simulink model "DSR_delay_beta_test"  (R2021a)
settings: Solver=VariableStepAuto  StartTime=0.0  StopTime=10  RelTol=1e-3
values from neighbouring files (symbols this model uses):
  a = 0    [gainMaxDef.m]    (also in plot2.m = 2; simulink_test.m = 5)
  alpha = 1.195    [gainMaxDef.m]    (also in plot2.m = 1.9; simulink_test.m = 1.192)
  betac = 2    [plot2.m]    (also in simulink_test.m = 10)
  c1 = 1    [simulink_test.m]
  delay = 0.5    [plot2.m]    (also in simulink_test.m = 0.015)
  delay_a = 0.150    (= 0.15)    [plot2.m]    (also in simulink_test.m = 0.01)
  gnet = 40    [plot2.m]    (also in simulink_test.m = gnetset(k))
  omega = omegalist(l)    [gainMaxDef.m]    (also in plot2.m = 300; simulink_test.m = 0.8)
  omegader = 80    [simulink_test.m]
undefined symbols (not defined in the file or in its folder): betacd
libraries: cstblocks x37, simulink x4
(part 3 of 3)

== system DSR_delay_beta_test/DSR_Input2/(I-beta*K)V_dot_est/DerivativeEstimate ==
  pos : Inport
  pos1 : Inport  Port=2
  pos2 : Inport  Port=3
  pos3 : Inport  Port=4
  pos4 : Inport  Port=5
  pos5 : Inport  Port=6
  Derivative Estimator : Subsystem
  Derivative Estimator1 : Subsystem
  Derivative Estimator2 : Subsystem
  Derivative Estimator3 : Subsystem
  Derivative Estimator4 : Subsystem
  Derivative Estimator5 : Subsystem
  est : Outport
  est1 : Outport  Port=2
  est2 : Outport  Port=3
  est3 : Outport  Port=4
  est4 : Outport  Port=5
  est5 : Outport  Port=6
  wires:
  pos3/1 -> Derivative Estimator3/1(pos)
  Derivative Estimator4/1(est) -> est4/1
  Derivative Estimator2/1(est) -> est2/1
  Derivative Estimator3/1(est) -> est3/1
  Derivative Estimator1/1(est) -> est1/1
  pos1/1 -> Derivative Estimator1/1(pos)
  Derivative Estimator5/1(est) -> est5/1
  Derivative Estimator/1(est) -> est/1
  pos/1 -> Derivative Estimator/1(pos)
  pos2/1 -> Derivative Estimator2/1(pos)
  pos5/1 -> Derivative Estimator5/1(pos)
  pos4/1 -> Derivative Estimator4/1(pos)

== system DSR_delay_beta_test/DSR_Input2/(I-beta*K)V_dot_est/DerivativeEstimate1 ==
  pos : Inport
  pos1 : Inport  Port=2
  pos2 : Inport  Port=3
  pos3 : Inport  Port=4
  pos4 : Inport  Port=5
  pos5 : Inport  Port=6
  Derivative Estimator : Subsystem
  Derivative Estimator1 : Subsystem
  Derivative Estimator2 : Subsystem
  Derivative Estimator3 : Subsystem
  Derivative Estimator4 : Subsystem
  Derivative Estimator5 : Subsystem
  est : Outport
  est1 : Outport  Port=2
  est2 : Outport  Port=3
  est3 : Outport  Port=4
  est4 : Outport  Port=5
  est5 : Outport  Port=6
  wires:
  pos3/1 -> Derivative Estimator3/1(pos)
  Derivative Estimator4/1(est) -> est4/1
  Derivative Estimator2/1(est) -> est2/1
  Derivative Estimator3/1(est) -> est3/1
  Derivative Estimator1/1(est) -> est1/1
  pos1/1 -> Derivative Estimator1/1(pos)
  Derivative Estimator5/1(est) -> est5/1
  Derivative Estimator/1(est) -> est/1
  pos/1 -> Derivative Estimator/1(pos)
  pos2/1 -> Derivative Estimator2/1(pos)
  pos5/1 -> Derivative Estimator5/1(pos)
  pos4/1 -> Derivative Estimator4/1(pos)

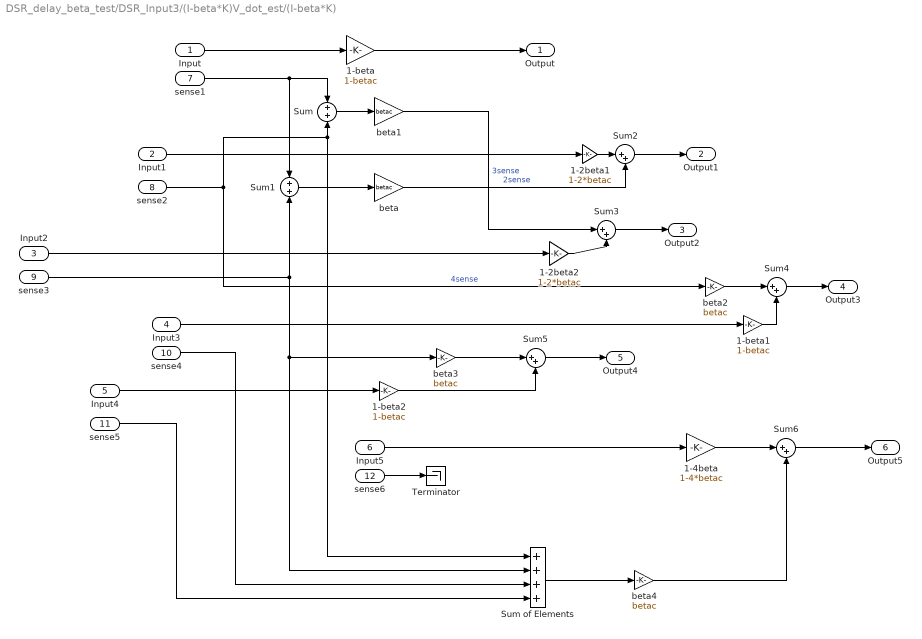
== system DSR_delay_beta_test/DSR_Input3/(I-beta*K)V_dot_est/(I-beta*K) ==
  Input : Inport
  Input1 : Inport  Port=2
  Input2 : Inport  Port=3
  Input3 : Inport  Port=4
  Input4 : Inport  Port=5
  Input5 : Inport  Port=6
  sense1 : Inport  Port=7
  sense2 : Inport  Port=8
  sense3 : Inport  Port=9
  sense4 : Inport  Port=10
  sense5 : Inport  Port=11
  sense6 : Inport  Port=12
  1-2beta1 : Gain  Gain=1-2*betac
  1-2beta2 : Gain  Gain=1-2*betac
  1-4beta : Gain  Gain=1-4*betac
  1-beta : Gain  Gain=1-betac
  1-beta1 : Gain  Gain=1-betac
  1-beta2 : Gain  Gain=1-betac
  Sum : Sum  Inputs=+|+
  Sum of Elements : Sum  Inputs=++++
  Sum1 : Sum  Inputs=+|+
  Sum{2..6} (5 alike) : Sum  Inputs=|++
  Terminator : Terminator
  beta{,1..4} (5 alike) : Gain  Gain=betac
  Output : Outport
  Output1 : Outport  Port=2
  Output2 : Outport  Port=3
  Output3 : Outport  Port=4
  Output4 : Outport  Port=5
  Output5 : Outport  Port=6
  wires:
  Input/1 -> 1-beta/1
  1-2beta2/1 -> Sum3/2
  1-beta2/1 -> Sum5/2
  Sum4/1 -> Output3/1
  1-beta/1 -> Output/1
  beta/1 -> Sum2/2  "2sense"
  Sum6/1 -> Output5/1
  1-beta1/1 -> Sum4/2
  Input2/1 -> 1-2beta2/1
  1-2beta1/1 -> Sum2/1
  Input1/1 -> 1-2beta1/1
  beta4/1 -> Sum6/2
  Sum/1 -> beta1/1
  Input3/1 -> 1-beta1/1
  beta3/1 -> Sum5/1
  beta1/1 -> Sum3/1  "3sense"
  beta2/1 -> Sum4/1
  Sum5/1 -> Output4/1
  Input4/1 -> 1-beta2/1
  Sum1/1 -> beta/1
  1-4beta/1 -> Sum6/1
  Sum2/1 -> Output1/1
  Sum3/1 -> Output2/1
  Input5/1 -> 1-4beta/1
  Sum of Elements/1 -> beta4/1
  sense1/1 -> Sum1/1, Sum/1
  sense2/1 -> beta2/1, Sum of Elements/1, Sum/2  "4sense"
  sense3/1 -> beta3/1, Sum of Elements/2, Sum1/2
  sense5/1 -> Sum of Elements/4
  sense4/1 -> Sum of Elements/3
  sense6/1 -> Terminator/1

== system DSR_delay_beta_test/DSR_Input3/(I-beta*K)V_dot_est/DerivativeEstimate ==
  pos : Inport
  pos1 : Inport  Port=2
  pos2 : Inport  Port=3
  pos3 : Inport  Port=4
  pos4 : Inport  Port=5
  pos5 : Inport  Port=6
  DSRdelayV1 : Subsystem
  DSRdelayV2 : Subsystem
  DSRdelayV3 : Subsystem
  DSRdelayV4 : Subsystem
  DSRdelayV5 : Subsystem
  DSRdelayV6 : Subsystem
  est : Outport
  est1 : Outport  Port=2
  est2 : Outport  Port=3
  est3 : Outport  Port=4
  est4 : Outport  Port=5
  est5 : Outport  Port=6
  wires:
  pos1/1 -> DSRdelayV1/1(Input)
  pos/1 -> DSRdelayV2/1(Input)
  DSRdelayV2/1(est) -> est/1
  pos2/1 -> DSRdelayV3/1(Input)
  pos3/1 -> DSRdelayV4/1(Input)
  pos4/1 -> DSRdelayV5/1(Input)
  pos5/1 -> DSRdelayV6/1(Input)
  DSRdelayV5/1(est) -> est4/1
  DSRdelayV6/1(est) -> est5/1
  DSRdelayV4/1(est) -> est3/1
  DSRdelayV3/1(est) -> est2/1
  DSRdelayV1/1(est) -> est1/1

== system DSR_delay_beta_test/DSR_Input3/(I-beta*K)V_dot_est/DerivativeEstimate1 ==
  pos : Inport
  pos1 : Inport  Port=2
  pos2 : Inport  Port=3
  pos3 : Inport  Port=4
  pos4 : Inport  Port=5
  pos5 : Inport  Port=6
  DSRdelayV1 : Subsystem
  DSRdelayV2 : Subsystem
  DSRdelayV3 : Subsystem
  DSRdelayV4 : Subsystem
  DSRdelayV5 : Subsystem
  DSRdelayV6 : Subsystem
  est : Outport
  est1 : Outport  Port=2
  est2 : Outport  Port=3
  est3 : Outport  Port=4
  est4 : Outport  Port=5
  est5 : Outport  Port=6
  wires:
  pos1/1 -> DSRdelayV1/1(Input)
  pos/1 -> DSRdelayV2/1(Input)
  DSRdelayV2/1(est) -> est/1
  pos2/1 -> DSRdelayV3/1(Input)
  pos3/1 -> DSRdelayV4/1(Input)
  pos4/1 -> DSRdelayV5/1(Input)
  pos5/1 -> DSRdelayV6/1(Input)
  DSRdelayV5/1(est) -> est4/1
  DSRdelayV6/1(est) -> est5/1
  DSRdelayV4/1(est) -> est3/1
  DSRdelayV3/1(est) -> est2/1
  DSRdelayV1/1(est) -> est1/1

== system DSR_delay_beta_test/DSR_Input1/(I-beta*K)V_dot_est/DerivativeEstimate/DSRdelayV1 ==
  Input : Inport
  Gain : Gain  Gain=1/delay
  Gain1 : Gain  Gain=1/delay
  Sum : Sum  Inputs=-+|
  Sum13 : Sum  Inputs=-+|
  Transfer Fcn : TransferFcn  Numerator=[omega]  Denominator=[1 omega]
  Transfer Fcn1 : TransferFcn  Numerator=[omega]  Denominator=[1 omega]
  Transport Delay : TransportDelay  DelayTime=delay
  Transport Delay13 : TransportDelay  DelayTime=delay
  est : Outport
  wires:
  Sum/1 -> Gain/1
  Gain/1 -> Transfer Fcn/1
  Transfer Fcn/1 -> Transport Delay13/1, Sum13/2
  Input/1 -> Transport Delay/1, Sum/2
  Transport Delay/1 -> Sum/1
  Transfer Fcn1/1 -> est/1
  Transport Delay13/1 -> Sum13/1
  Gain1/1 -> Transfer Fcn1/1
  Sum13/1 -> Gain1/1

== system DSR_delay_beta_test/DSR_Input1/(I-beta*K)V_dot_est/DerivativeEstimate/DSRdelayV2 ==
  Input : Inport
  Gain : Gain  Gain=1/delay
  Gain1 : Gain  Gain=1/delay
  Sum : Sum  Inputs=-+|
  Sum13 : Sum  Inputs=-+|
  Transfer Fcn : TransferFcn  Numerator=[omega]  Denominator=[1 omega]
  Transfer Fcn1 : TransferFcn  Numerator=[omega]  Denominator=[1 omega]
  Transport Delay : TransportDelay  DelayTime=delay
  Transport Delay13 : TransportDelay  DelayTime=delay
  est : Outport
  wires:
  Sum/1 -> Gain/1
  Gain/1 -> Transfer Fcn/1
  Transfer Fcn/1 -> Transport Delay13/1, Sum13/2
  Input/1 -> Transport Delay/1, Sum/2
  Transport Delay/1 -> Sum/1
  Transfer Fcn1/1 -> est/1
  Transport Delay13/1 -> Sum13/1
  Gain1/1 -> Transfer Fcn1/1
  Sum13/1 -> Gain1/1

== system DSR_delay_beta_test/DSR_Input1/(I-beta*K)V_dot_est/DerivativeEstimate/DSRdelayV3 ==
  Input : Inport
  Gain : Gain  Gain=1/delay
  Gain1 : Gain  Gain=1/delay
  Sum : Sum  Inputs=-+|
  Sum13 : Sum  Inputs=-+|
  Transfer Fcn : TransferFcn  Numerator=[omega]  Denominator=[1 omega]
  Transfer Fcn1 : TransferFcn  Numerator=[omega]  Denominator=[1 omega]
  Transport Delay : TransportDelay  DelayTime=delay
  Transport Delay13 : TransportDelay  DelayTime=delay
  est : Outport
  wires:
  Sum/1 -> Gain/1
  Gain/1 -> Transfer Fcn/1
  Transfer Fcn/1 -> Transport Delay13/1, Sum13/2
  Input/1 -> Transport Delay/1, Sum/2
  Transport Delay/1 -> Sum/1
  Transfer Fcn1/1 -> est/1
  Transport Delay13/1 -> Sum13/1
  Gain1/1 -> Transfer Fcn1/1
  Sum13/1 -> Gain1/1

== system DSR_delay_beta_test/DSR_Input1/(I-beta*K)V_dot_est/DerivativeEstimate/DSRdelayV4 ==
  Input : Inport
  Gain : Gain  Gain=1/delay
  Gain1 : Gain  Gain=1/delay
  Sum : Sum  Inputs=-+|
  Sum13 : Sum  Inputs=-+|
  Transfer Fcn : TransferFcn  Numerator=[omega]  Denominator=[1 omega]
  Transfer Fcn1 : TransferFcn  Numerator=[omega]  Denominator=[1 omega]
  Transport Delay : TransportDelay  DelayTime=delay
  Transport Delay13 : TransportDelay  DelayTime=delay
  est : Outport
  wires:
  Sum/1 -> Gain/1
  Gain/1 -> Transfer Fcn/1
  Transfer Fcn/1 -> Transport Delay13/1, Sum13/2
  Input/1 -> Transport Delay/1, Sum/2
  Transport Delay/1 -> Sum/1
  Transfer Fcn1/1 -> est/1
  Transport Delay13/1 -> Sum13/1
  Gain1/1 -> Transfer Fcn1/1
  Sum13/1 -> Gain1/1

== system DSR_delay_beta_test/DSR_Input1/(I-beta*K)V_dot_est/DerivativeEstimate/DSRdelayV5 ==
  Input : Inport
  Gain : Gain  Gain=1/delay
  Gain1 : Gain  Gain=1/delay
  Sum : Sum  Inputs=-+|
  Sum13 : Sum  Inputs=-+|
  Transfer Fcn : TransferFcn  Numerator=[omega]  Denominator=[1 omega]
  Transfer Fcn1 : TransferFcn  Numerator=[omega]  Denominator=[1 omega]
  Transport Delay : TransportDelay  DelayTime=delay
  Transport Delay13 : TransportDelay  DelayTime=delay
  est : Outport
  wires:
  Sum/1 -> Gain/1
  Gain/1 -> Transfer Fcn/1
  Transfer Fcn/1 -> Transport Delay13/1, Sum13/2
  Input/1 -> Transport Delay/1, Sum/2
  Transport Delay/1 -> Sum/1
  Transfer Fcn1/1 -> est/1
  Transport Delay13/1 -> Sum13/1
  Gain1/1 -> Transfer Fcn1/1
  Sum13/1 -> Gain1/1

== system DSR_delay_beta_test/DSR_Input1/(I-beta*K)V_dot_est/DerivativeEstimate/DSRdelayV6 ==
  Input : Inport
  Gain : Gain  Gain=1/delay
  Gain1 : Gain  Gain=1/delay
  Sum : Sum  Inputs=-+|
  Sum13 : Sum  Inputs=-+|
  Transfer Fcn : TransferFcn  Numerator=[omega]  Denominator=[1 omega]
  Transfer Fcn1 : TransferFcn  Numerator=[omega]  Denominator=[1 omega]
  Transport Delay : TransportDelay  DelayTime=delay
  Transport Delay13 : TransportDelay  DelayTime=delay
  est : Outport
  wires:
  Sum/1 -> Gain/1
  Gain/1 -> Transfer Fcn/1
  Transfer Fcn/1 -> Transport Delay13/1, Sum13/2
  Input/1 -> Transport Delay/1, Sum/2
  Transport Delay/1 -> Sum/1
  Transfer Fcn1/1 -> est/1
  Transport Delay13/1 -> Sum13/1
  Gain1/1 -> Transfer Fcn1/1
  Sum13/1 -> Gain1/1

== system DSR_delay_beta_test/DSR_Input1/(I-beta*K)V_dot_est/DerivativeEstimate1/DSRdelayV1 ==
  Input : Inport
  Gain : Gain  Gain=1/delay
  Gain1 : Gain  Gain=1/delay
  Sum : Sum  Inputs=-+|
  Sum13 : Sum  Inputs=-+|
  Transfer Fcn : TransferFcn  Numerator=[omega]  Denominator=[1 omega]
  Transfer Fcn1 : TransferFcn  Numerator=[omega]  Denominator=[1 omega]
  Transport Delay : TransportDelay  DelayTime=delay
  Transport Delay13 : TransportDelay  DelayTime=delay
  est : Outport
  wires:
  Sum/1 -> Gain/1
  Gain/1 -> Transfer Fcn/1
  Transfer Fcn/1 -> Transport Delay13/1, Sum13/2
  Input/1 -> Transport Delay/1, Sum/2
  Transport Delay/1 -> Sum/1
  Transfer Fcn1/1 -> est/1
  Transport Delay13/1 -> Sum13/1
  Gain1/1 -> Transfer Fcn1/1
  Sum13/1 -> Gain1/1

== system DSR_delay_beta_test/DSR_Input1/(I-beta*K)V_dot_est/DerivativeEstimate1/DSRdelayV2 ==
  Input : Inport
  Gain : Gain  Gain=1/delay
  Gain1 : Gain  Gain=1/delay
  Scope : Scope  NumInputPorts=5
  Sum : Sum  Inputs=-+|
  Sum13 : Sum  Inputs=-+|
  Transfer Fcn : TransferFcn  Numerator=[omega]  Denominator=[1 omega]
  Transfer Fcn1 : TransferFcn  Numerator=[omega]  Denominator=[1 omega]
  Transport Delay : TransportDelay  DelayTime=delay
  Transport Delay13 : TransportDelay  DelayTime=delay
  est : Outport
  wires:
  Sum/1 -> Gain/1
  Gain/1 -> Scope/2, Transfer Fcn/1
  Transfer Fcn/1 -> Transport Delay13/1, Sum13/2, Scope/3
  Input/1 -> Transport Delay/1, Scope/1, Sum/2
  Transport Delay/1 -> Sum/1
  Transfer Fcn1/1 -> Scope/5, est/1
  Transport Delay13/1 -> Sum13/1
  Gain1/1 -> Scope/4, Transfer Fcn1/1
  Sum13/1 -> Gain1/1

== system DSR_delay_beta_test/DSR_Input1/(I-beta*K)V_dot_est/DerivativeEstimate1/DSRdelayV3 ==
  Input : Inport
  Gain : Gain  Gain=1/delay
  Gain1 : Gain  Gain=1/delay
  Sum : Sum  Inputs=-+|
  Sum13 : Sum  Inputs=-+|
  Transfer Fcn : TransferFcn  Numerator=[omega]  Denominator=[1 omega]
  Transfer Fcn1 : TransferFcn  Numerator=[omega]  Denominator=[1 omega]
  Transport Delay : TransportDelay  DelayTime=delay
  Transport Delay13 : TransportDelay  DelayTime=delay
  est : Outport
  wires:
  Sum/1 -> Gain/1
  Gain/1 -> Transfer Fcn/1
  Transfer Fcn/1 -> Transport Delay13/1, Sum13/2
  Input/1 -> Transport Delay/1, Sum/2
  Transport Delay/1 -> Sum/1
  Transfer Fcn1/1 -> est/1
  Transport Delay13/1 -> Sum13/1
  Gain1/1 -> Transfer Fcn1/1
  Sum13/1 -> Gain1/1

== system DSR_delay_beta_test/DSR_Input1/(I-beta*K)V_dot_est/DerivativeEstimate1/DSRdelayV4 ==
  Input : Inport
  Gain : Gain  Gain=1/delay
  Gain1 : Gain  Gain=1/delay
  Sum : Sum  Inputs=-+|
  Sum13 : Sum  Inputs=-+|
  Transfer Fcn : TransferFcn  Numerator=[omega]  Denominator=[1 omega]
  Transfer Fcn1 : TransferFcn  Numerator=[omega]  Denominator=[1 omega]
  Transport Delay : TransportDelay  DelayTime=delay
  Transport Delay13 : TransportDelay  DelayTime=delay
  est : Outport
  wires:
  Sum/1 -> Gain/1
  Gain/1 -> Transfer Fcn/1
  Transfer Fcn/1 -> Transport Delay13/1, Sum13/2
  Input/1 -> Transport Delay/1, Sum/2
  Transport Delay/1 -> Sum/1
  Transfer Fcn1/1 -> est/1
  Transport Delay13/1 -> Sum13/1
  Gain1/1 -> Transfer Fcn1/1
  Sum13/1 -> Gain1/1

== system DSR_delay_beta_test/DSR_Input1/(I-beta*K)V_dot_est/DerivativeEstimate1/DSRdelayV5 ==
  Input : Inport
  Gain : Gain  Gain=1/delay
  Gain1 : Gain  Gain=1/delay
  Sum : Sum  Inputs=-+|
  Sum13 : Sum  Inputs=-+|
  Transfer Fcn : TransferFcn  Numerator=[omega]  Denominator=[1 omega]
  Transfer Fcn1 : TransferFcn  Numerator=[omega]  Denominator=[1 omega]
  Transport Delay : TransportDelay  DelayTime=delay
  Transport Delay13 : TransportDelay  DelayTime=delay
  est : Outport
  wires:
  Sum/1 -> Gain/1
  Gain/1 -> Transfer Fcn/1
  Transfer Fcn/1 -> Transport Delay13/1, Sum13/2
  Input/1 -> Transport Delay/1, Sum/2
  Transport Delay/1 -> Sum/1
  Transfer Fcn1/1 -> est/1
  Transport Delay13/1 -> Sum13/1
  Gain1/1 -> Transfer Fcn1/1
  Sum13/1 -> Gain1/1

== system DSR_delay_beta_test/DSR_Input1/(I-beta*K)V_dot_est/DerivativeEstimate1/DSRdelayV6 ==
  Input : Inport
  Gain : Gain  Gain=1/delay
  Gain1 : Gain  Gain=1/delay
  Sum : Sum  Inputs=-+|
  Sum13 : Sum  Inputs=-+|
  Transfer Fcn : TransferFcn  Numerator=[omega]  Denominator=[1 omega]
  Transfer Fcn1 : TransferFcn  Numerator=[omega]  Denominator=[1 omega]
  Transport Delay : TransportDelay  DelayTime=delay
  Transport Delay13 : TransportDelay  DelayTime=delay
  est : Outport
  wires:
  Sum/1 -> Gain/1
  Gain/1 -> Transfer Fcn/1
  Transfer Fcn/1 -> Transport Delay13/1, Sum13/2
  Input/1 -> Transport Delay/1, Sum/2
  Transport Delay/1 -> Sum/1
  Transfer Fcn1/1 -> est/1
  Transport Delay13/1 -> Sum13/1
  Gain1/1 -> Transfer Fcn1/1
  Sum13/1 -> Gain1/1

== system DSR_delay_beta_test/DSR_Input2/(I-beta*K)V_dot_est/DerivativeEstimate/Derivative Estimator ==
  pos : Inport
  DSRdelay : Subsystem
  LPF : TransferFcn  Numerator=[omega^2]  Denominator=[delay^2 2*omega*delay^2 omega^2*delay^2]
  est : Outport
  wires:
  LPF/1 -> DSRdelay/1(Input)
  DSRdelay/1(Out1) -> est/1
  pos/1 -> LPF/1

== system DSR_delay_beta_test/DSR_Input2/(I-beta*K)V_dot_est/DerivativeEstimate/Derivative Estimator1 ==
  pos : Inport
  DSRdelay : Subsystem
  LPF : TransferFcn  Numerator=[omega^2]  Denominator=[delay^2 2*omega*delay^2 omega^2*delay^2]
  est : Outport
  wires:
  LPF/1 -> DSRdelay/1(Input)
  DSRdelay/1(Out1) -> est/1
  pos/1 -> LPF/1

== system DSR_delay_beta_test/DSR_Input2/(I-beta*K)V_dot_est/DerivativeEstimate/Derivative Estimator2 ==
  pos : Inport
  DSRdelay : Subsystem
  LPF : TransferFcn  Numerator=[omega^2]  Denominator=[delay^2 2*omega*delay^2 omega^2*delay^2]
  est : Outport
  wires:
  LPF/1 -> DSRdelay/1(Input)
  DSRdelay/1(Out1) -> est/1
  pos/1 -> LPF/1

== system DSR_delay_beta_test/DSR_Input2/(I-beta*K)V_dot_est/DerivativeEstimate/Derivative Estimator3 ==
  pos : Inport
  DSRdelay : Subsystem
  LPF : TransferFcn  Numerator=[omega^2]  Denominator=[delay^2 2*omega*delay^2 omega^2*delay^2]
  est : Outport
  wires:
  LPF/1 -> DSRdelay/1(Input)
  DSRdelay/1(Out1) -> est/1
  pos/1 -> LPF/1

== system DSR_delay_beta_test/DSR_Input2/(I-beta*K)V_dot_est/DerivativeEstimate/Derivative Estimator4 ==
  pos : Inport
  DSRdelay : Subsystem
  LPF : TransferFcn  Numerator=[omega^2]  Denominator=[delay^2 2*omega*delay^2 omega^2*delay^2]
  est : Outport
  wires:
  LPF/1 -> DSRdelay/1(Input)
  DSRdelay/1(Out1) -> est/1
  pos/1 -> LPF/1

== system DSR_delay_beta_test/DSR_Input2/(I-beta*K)V_dot_est/DerivativeEstimate/Derivative Estimator5 ==
  pos : Inport
  DSRdelay : Subsystem
  LPF : TransferFcn  Numerator=[omega^2]  Denominator=[delay^2 2*omega*delay^2 omega^2*delay^2]
  est : Outport
  wires:
  LPF/1 -> DSRdelay/1(Input)
  DSRdelay/1(Out1) -> est/1
  pos/1 -> LPF/1

== system DSR_delay_beta_test/DSR_Input2/(I-beta*K)V_dot_est/DerivativeEstimate1/Derivative Estimator ==
  pos : Inport
  DSRdelay : Subsystem
  LPF : TransferFcn  Numerator=[omega^2]  Denominator=[delay^2 2*omega*delay^2 omega^2*delay^2]
  est : Outport
  wires:
  LPF/1 -> DSRdelay/1(Input)
  DSRdelay/1(Out1) -> est/1
  pos/1 -> LPF/1

== system DSR_delay_beta_test/DSR_Input2/(I-beta*K)V_dot_est/DerivativeEstimate1/Derivative Estimator1 ==
  pos : Inport
  DSRdelay : Subsystem
  LPF : TransferFcn  Numerator=[omega^2]  Denominator=[delay^2 2*omega*delay^2 omega^2*delay^2]
  est : Outport
  wires:
  LPF/1 -> DSRdelay/1(Input)
  DSRdelay/1(Out1) -> est/1
  pos/1 -> LPF/1

== system DSR_delay_beta_test/DSR_Input2/(I-beta*K)V_dot_est/DerivativeEstimate1/Derivative Estimator2 ==
  pos : Inport
  DSRdelay : Subsystem
  LPF : TransferFcn  Numerator=[omega^2]  Denominator=[delay^2 2*omega*delay^2 omega^2*delay^2]
  est : Outport
  wires:
  LPF/1 -> DSRdelay/1(Input)
  DSRdelay/1(Out1) -> est/1
  pos/1 -> LPF/1

== system DSR_delay_beta_test/DSR_Input2/(I-beta*K)V_dot_est/DerivativeEstimate1/Derivative Estimator3 ==
  pos : Inport
  DSRdelay : Subsystem
  LPF : TransferFcn  Numerator=[omega^2]  Denominator=[delay^2 2*omega*delay^2 omega^2*delay^2]
  est : Outport
  wires:
  LPF/1 -> DSRdelay/1(Input)
  DSRdelay/1(Out1) -> est/1
  pos/1 -> LPF/1

== system DSR_delay_beta_test/DSR_Input2/(I-beta*K)V_dot_est/DerivativeEstimate1/Derivative Estimator4 ==
  pos : Inport
  DSRdelay : Subsystem
  LPF : TransferFcn  Numerator=[omega^2]  Denominator=[delay^2 2*omega*delay^2 omega^2*delay^2]
  est : Outport
  wires:
  LPF/1 -> DSRdelay/1(Input)
  DSRdelay/1(Out1) -> est/1
  pos/1 -> LPF/1

== system DSR_delay_beta_test/DSR_Input2/(I-beta*K)V_dot_est/DerivativeEstimate1/Derivative Estimator5 ==
  pos : Inport
  DSRdelay : Subsystem
  LPF : TransferFcn  Numerator=[omega^2]  Denominator=[delay^2 2*omega*delay^2 omega^2*delay^2]
  est : Outport
  wires:
  LPF/1 -> DSRdelay/1(Input)
  DSRdelay/1(Out1) -> est/1
  pos/1 -> LPF/1

== system DSR_delay_beta_test/DSR_Input3/(I-beta*K)V_dot_est/DerivativeEstimate/DSRdelayV1 ==
  Input : Inport
  Gain : Gain  Gain=1/delay
  Gain1 : Gain  Gain=1/delay
  Sum : Sum  Inputs=-+|
  Sum13 : Sum  Inputs=-+|
  Transfer Fcn : TransferFcn  Numerator=[omega]  Denominator=[1 omega]
  Transfer Fcn1 : TransferFcn  Numerator=[omega]  Denominator=[1 omega]
  Transport Delay : TransportDelay  DelayTime=delay
  Transport Delay13 : TransportDelay  DelayTime=delay
  est : Outport
  wires:
  Sum/1 -> Gain/1
  Gain/1 -> Transfer Fcn/1
  Transfer Fcn/1 -> Transport Delay13/1, Sum13/2
  Input/1 -> Transport Delay/1, Sum/2
  Transport Delay/1 -> Sum/1
  Transfer Fcn1/1 -> est/1
  Transport Delay13/1 -> Sum13/1
  Gain1/1 -> Transfer Fcn1/1
  Sum13/1 -> Gain1/1

== system DSR_delay_beta_test/DSR_Input3/(I-beta*K)V_dot_est/DerivativeEstimate/DSRdelayV2 ==
  Input : Inport
  Gain : Gain  Gain=1/delay
  Gain1 : Gain  Gain=1/delay
  Sum : Sum  Inputs=-+|
  Sum13 : Sum  Inputs=-+|
  Transfer Fcn : TransferFcn  Numerator=[omega]  Denominator=[1 omega]
  Transfer Fcn1 : TransferFcn  Numerator=[omega]  Denominator=[1 omega]
  Transport Delay : TransportDelay  DelayTime=delay
  Transport Delay13 : TransportDelay  DelayTime=delay
  est : Outport
  wires:
  Sum/1 -> Gain/1
  Gain/1 -> Transfer Fcn/1
  Transfer Fcn/1 -> Transport Delay13/1, Sum13/2
  Input/1 -> Transport Delay/1, Sum/2
  Transport Delay/1 -> Sum/1
  Transfer Fcn1/1 -> est/1
  Transport Delay13/1 -> Sum13/1
  Gain1/1 -> Transfer Fcn1/1
  Sum13/1 -> Gain1/1

== system DSR_delay_beta_test/DSR_Input3/(I-beta*K)V_dot_est/DerivativeEstimate/DSRdelayV3 ==
  Input : Inport
  Gain : Gain  Gain=1/delay
  Gain1 : Gain  Gain=1/delay
  Sum : Sum  Inputs=-+|
  Sum13 : Sum  Inputs=-+|
  Transfer Fcn : TransferFcn  Numerator=[omega]  Denominator=[1 omega]
  Transfer Fcn1 : TransferFcn  Numerator=[omega]  Denominator=[1 omega]
  Transport Delay : TransportDelay  DelayTime=delay
  Transport Delay13 : TransportDelay  DelayTime=delay
  est : Outport
  wires:
  Sum/1 -> Gain/1
  Gain/1 -> Transfer Fcn/1
  Transfer Fcn/1 -> Transport Delay13/1, Sum13/2
  Input/1 -> Transport Delay/1, Sum/2
  Transport Delay/1 -> Sum/1
  Transfer Fcn1/1 -> est/1
  Transport Delay13/1 -> Sum13/1
  Gain1/1 -> Transfer Fcn1/1
  Sum13/1 -> Gain1/1

== system DSR_delay_beta_test/DSR_Input3/(I-beta*K)V_dot_est/DerivativeEstimate/DSRdelayV4 ==
  Input : Inport
  Gain : Gain  Gain=1/delay
  Gain1 : Gain  Gain=1/delay
  Sum : Sum  Inputs=-+|
  Sum13 : Sum  Inputs=-+|
  Transfer Fcn : TransferFcn  Numerator=[omega]  Denominator=[1 omega]
  Transfer Fcn1 : TransferFcn  Numerator=[omega]  Denominator=[1 omega]
  Transport Delay : TransportDelay  DelayTime=delay
  Transport Delay13 : TransportDelay  DelayTime=delay
  est : Outport
  wires:
  Sum/1 -> Gain/1
  Gain/1 -> Transfer Fcn/1
  Transfer Fcn/1 -> Transport Delay13/1, Sum13/2
  Input/1 -> Transport Delay/1, Sum/2
  Transport Delay/1 -> Sum/1
  Transfer Fcn1/1 -> est/1
  Transport Delay13/1 -> Sum13/1
  Gain1/1 -> Transfer Fcn1/1
  Sum13/1 -> Gain1/1

== system DSR_delay_beta_test/DSR_Input3/(I-beta*K)V_dot_est/DerivativeEstimate/DSRdelayV5 ==
  Input : Inport
  Gain : Gain  Gain=1/delay
  Gain1 : Gain  Gain=1/delay
  Sum : Sum  Inputs=-+|
  Sum13 : Sum  Inputs=-+|
  Transfer Fcn : TransferFcn  Numerator=[omega]  Denominator=[1 omega]
  Transfer Fcn1 : TransferFcn  Numerator=[omega]  Denominator=[1 omega]
  Transport Delay : TransportDelay  DelayTime=delay
  Transport Delay13 : TransportDelay  DelayTime=delay
  est : Outport
  wires:
  Sum/1 -> Gain/1
  Gain/1 -> Transfer Fcn/1
  Transfer Fcn/1 -> Transport Delay13/1, Sum13/2
  Input/1 -> Transport Delay/1, Sum/2
  Transport Delay/1 -> Sum/1
  Transfer Fcn1/1 -> est/1
  Transport Delay13/1 -> Sum13/1
  Gain1/1 -> Transfer Fcn1/1
  Sum13/1 -> Gain1/1

== system DSR_delay_beta_test/DSR_Input3/(I-beta*K)V_dot_est/DerivativeEstimate/DSRdelayV6 ==
  Input : Inport
  Gain : Gain  Gain=1/delay
  Gain1 : Gain  Gain=1/delay
  Sum : Sum  Inputs=-+|
  Sum13 : Sum  Inputs=-+|
  Transfer Fcn : TransferFcn  Numerator=[omega]  Denominator=[1 omega]
  Transfer Fcn1 : TransferFcn  Numerator=[omega]  Denominator=[1 omega]
  Transport Delay : TransportDelay  DelayTime=delay
  Transport Delay13 : TransportDelay  DelayTime=delay
  est : Outport
  wires:
  Sum/1 -> Gain/1
  Gain/1 -> Transfer Fcn/1
  Transfer Fcn/1 -> Transport Delay13/1, Sum13/2
  Input/1 -> Transport Delay/1, Sum/2
  Transport Delay/1 -> Sum/1
  Transfer Fcn1/1 -> est/1
  Transport Delay13/1 -> Sum13/1
  Gain1/1 -> Transfer Fcn1/1
  Sum13/1 -> Gain1/1

== system DSR_delay_beta_test/DSR_Input3/(I-beta*K)V_dot_est/DerivativeEstimate1/DSRdelayV1 ==
  Input : Inport
  Gain : Gain  Gain=1/delay
  Gain1 : Gain  Gain=1/delay
  Sum : Sum  Inputs=-+|
  Sum13 : Sum  Inputs=-+|
  Transfer Fcn : TransferFcn  Numerator=[omega]  Denominator=[1 omega]
  Transfer Fcn1 : TransferFcn  Numerator=[omega]  Denominator=[1 omega]
  Transport Delay : TransportDelay  DelayTime=delay
  Transport Delay13 : TransportDelay  DelayTime=delay
  est : Outport
  wires:
  Sum/1 -> Gain/1
  Gain/1 -> Transfer Fcn/1
  Transfer Fcn/1 -> Transport Delay13/1, Sum13/2
  Input/1 -> Transport Delay/1, Sum/2
  Transport Delay/1 -> Sum/1
  Transfer Fcn1/1 -> est/1
  Transport Delay13/1 -> Sum13/1
  Gain1/1 -> Transfer Fcn1/1
  Sum13/1 -> Gain1/1

== system DSR_delay_beta_test/DSR_Input3/(I-beta*K)V_dot_est/DerivativeEstimate1/DSRdelayV2 ==
  Input : Inport
  Gain : Gain  Gain=1/delay
  Gain1 : Gain  Gain=1/delay
  Scope : Scope  NumInputPorts=5
  Sum : Sum  Inputs=-+|
  Sum13 : Sum  Inputs=-+|
  Transfer Fcn : TransferFcn  Numerator=[omega]  Denominator=[1 omega]
  Transfer Fcn1 : TransferFcn  Numerator=[omega]  Denominator=[1 omega]
  Transport Delay : TransportDelay  DelayTime=delay
  Transport Delay13 : TransportDelay  DelayTime=delay
  est : Outport
  wires:
  Sum/1 -> Gain/1
  Gain/1 -> Scope/2, Transfer Fcn/1
  Transfer Fcn/1 -> Transport Delay13/1, Sum13/2, Scope/3
  Input/1 -> Transport Delay/1, Scope/1, Sum/2
  Transport Delay/1 -> Sum/1
  Transfer Fcn1/1 -> Scope/5, est/1
  Transport Delay13/1 -> Sum13/1
  Gain1/1 -> Scope/4, Transfer Fcn1/1
  Sum13/1 -> Gain1/1

== system DSR_delay_beta_test/DSR_Input3/(I-beta*K)V_dot_est/DerivativeEstimate1/DSRdelayV3 ==
  Input : Inport
  Gain : Gain  Gain=1/delay
  Gain1 : Gain  Gain=1/delay
  Sum : Sum  Inputs=-+|
  Sum13 : Sum  Inputs=-+|
  Transfer Fcn : TransferFcn  Numerator=[omega]  Denominator=[1 omega]
  Transfer Fcn1 : TransferFcn  Numerator=[omega]  Denominator=[1 omega]
  Transport Delay : TransportDelay  DelayTime=delay
  Transport Delay13 : TransportDelay  DelayTime=delay
  est : Outport
  wires:
  Sum/1 -> Gain/1
  Gain/1 -> Transfer Fcn/1
  Transfer Fcn/1 -> Transport Delay13/1, Sum13/2
  Input/1 -> Transport Delay/1, Sum/2
  Transport Delay/1 -> Sum/1
  Transfer Fcn1/1 -> est/1
  Transport Delay13/1 -> Sum13/1
  Gain1/1 -> Transfer Fcn1/1
  Sum13/1 -> Gain1/1

== system DSR_delay_beta_test/DSR_Input3/(I-beta*K)V_dot_est/DerivativeEstimate1/DSRdelayV4 ==
  Input : Inport
  Gain : Gain  Gain=1/delay
  Gain1 : Gain  Gain=1/delay
  Sum : Sum  Inputs=-+|
  Sum13 : Sum  Inputs=-+|
  Transfer Fcn : TransferFcn  Numerator=[omega]  Denominator=[1 omega]
  Transfer Fcn1 : TransferFcn  Numerator=[omega]  Denominator=[1 omega]
  Transport Delay : TransportDelay  DelayTime=delay
  Transport Delay13 : TransportDelay  DelayTime=delay
  est : Outport
  wires:
  Sum/1 -> Gain/1
  Gain/1 -> Transfer Fcn/1
  Transfer Fcn/1 -> Transport Delay13/1, Sum13/2
  Input/1 -> Transport Delay/1, Sum/2
  Transport Delay/1 -> Sum/1
  Transfer Fcn1/1 -> est/1
  Transport Delay13/1 -> Sum13/1
  Gain1/1 -> Transfer Fcn1/1
  Sum13/1 -> Gain1/1

== system DSR_delay_beta_test/DSR_Input3/(I-beta*K)V_dot_est/DerivativeEstimate1/DSRdelayV5 ==
  Input : Inport
  Gain : Gain  Gain=1/delay
  Gain1 : Gain  Gain=1/delay
  Sum : Sum  Inputs=-+|
  Sum13 : Sum  Inputs=-+|
  Transfer Fcn : TransferFcn  Numerator=[omega]  Denominator=[1 omega]
  Transfer Fcn1 : TransferFcn  Numerator=[omega]  Denominator=[1 omega]
  Transport Delay : TransportDelay  DelayTime=delay
  Transport Delay13 : TransportDelay  DelayTime=delay
  est : Outport
  wires:
  Sum/1 -> Gain/1
  Gain/1 -> Transfer Fcn/1
  Transfer Fcn/1 -> Transport Delay13/1, Sum13/2
  Input/1 -> Transport Delay/1, Sum/2
  Transport Delay/1 -> Sum/1
  Transfer Fcn1/1 -> est/1
  Transport Delay13/1 -> Sum13/1
  Gain1/1 -> Transfer Fcn1/1
  Sum13/1 -> Gain1/1

== system DSR_delay_beta_test/DSR_Input3/(I-beta*K)V_dot_est/DerivativeEstimate1/DSRdelayV6 ==
  Input : Inport
  Gain : Gain  Gain=1/delay
  Gain1 : Gain  Gain=1/delay
  Sum : Sum  Inputs=-+|
  Sum13 : Sum  Inputs=-+|
  Transfer Fcn : TransferFcn  Numerator=[omega]  Denominator=[1 omega]
  Transfer Fcn1 : TransferFcn  Numerator=[omega]  Denominator=[1 omega]
  Transport Delay : TransportDelay  DelayTime=delay
  Transport Delay13 : TransportDelay  DelayTime=delay
  est : Outport
  wires:
  Sum/1 -> Gain/1
  Gain/1 -> Transfer Fcn/1
  Transfer Fcn/1 -> Transport Delay13/1, Sum13/2
  Input/1 -> Transport Delay/1, Sum/2
  Transport Delay/1 -> Sum/1
  Transfer Fcn1/1 -> est/1
  Transport Delay13/1 -> Sum13/1
  Gain1/1 -> Transfer Fcn1/1
  Sum13/1 -> Gain1/1

== system DSR_delay_beta_test/DSR_Input2/(I-beta*K)V_dot_est/DerivativeEstimate/Derivative Estimator/DSRdelay ==
  Input : Inport
  Gain : Gain  Gain=2
  Sum : Sum  Inputs=-++
  Transport Delay1 : TransportDelay  DelayTime=2*delay
  Transport Delay2 : TransportDelay  DelayTime=delay
  Out1 : Outport
  wires:
  Input/1 -> Transport Delay2/1, Transport Delay1/1, Sum/2
  Transport Delay2/1 -> Gain/1
  Transport Delay1/1 -> Sum/3
  Gain/1 -> Sum/1
  Sum/1 -> Out1/1

== system DSR_delay_beta_test/DSR_Input2/(I-beta*K)V_dot_est/DerivativeEstimate/Derivative Estimator1/DSRdelay ==
  Input : Inport
  Gain : Gain  Gain=2
  Sum : Sum  Inputs=-++
  Transport Delay1 : TransportDelay  DelayTime=2*delay
  Transport Delay2 : TransportDelay  DelayTime=delay
  Out1 : Outport
  wires:
  Input/1 -> Transport Delay2/1, Transport Delay1/1, Sum/2
  Transport Delay2/1 -> Gain/1
  Transport Delay1/1 -> Sum/3
  Gain/1 -> Sum/1
  Sum/1 -> Out1/1

== system DSR_delay_beta_test/DSR_Input2/(I-beta*K)V_dot_est/DerivativeEstimate/Derivative Estimator2/DSRdelay ==
  Input : Inport
  Gain : Gain  Gain=2
  Sum : Sum  Inputs=-++
  Transport Delay1 : TransportDelay  DelayTime=2*delay
  Transport Delay2 : TransportDelay  DelayTime=delay
  Out1 : Outport
  wires:
  Input/1 -> Transport Delay2/1, Transport Delay1/1, Sum/2
  Transport Delay2/1 -> Gain/1
  Transport Delay1/1 -> Sum/3
  Gain/1 -> Sum/1
  Sum/1 -> Out1/1

== system DSR_delay_beta_test/DSR_Input2/(I-beta*K)V_dot_est/DerivativeEstimate/Derivative Estimator3/DSRdelay ==
  Input : Inport
  Gain : Gain  Gain=2
  Sum : Sum  Inputs=-++
  Transport Delay1 : TransportDelay  DelayTime=2*delay
  Transport Delay2 : TransportDelay  DelayTime=delay
  Out1 : Outport
  wires:
  Input/1 -> Transport Delay2/1, Transport Delay1/1, Sum/2
  Transport Delay2/1 -> Gain/1
  Transport Delay1/1 -> Sum/3
  Gain/1 -> Sum/1
  Sum/1 -> Out1/1

== system DSR_delay_beta_test/DSR_Input2/(I-beta*K)V_dot_est/DerivativeEstimate/Derivative Estimator4/DSRdelay ==
  Input : Inport
  Gain : Gain  Gain=2
  Sum : Sum  Inputs=-++
  Transport Delay1 : TransportDelay  DelayTime=2*delay
  Transport Delay2 : TransportDelay  DelayTime=delay
  Out1 : Outport
  wires:
  Input/1 -> Transport Delay2/1, Transport Delay1/1, Sum/2
  Transport Delay2/1 -> Gain/1
  Transport Delay1/1 -> Sum/3
  Gain/1 -> Sum/1
  Sum/1 -> Out1/1

== system DSR_delay_beta_test/DSR_Input2/(I-beta*K)V_dot_est/DerivativeEstimate/Derivative Estimator5/DSRdelay ==
  Input : Inport
  Gain : Gain  Gain=2
  Sum : Sum  Inputs=-++
  Transport Delay1 : TransportDelay  DelayTime=2*delay
  Transport Delay2 : TransportDelay  DelayTime=delay
  Out1 : Outport
  wires:
  Input/1 -> Transport Delay2/1, Transport Delay1/1, Sum/2
  Transport Delay2/1 -> Gain/1
  Transport Delay1/1 -> Sum/3
  Gain/1 -> Sum/1
  Sum/1 -> Out1/1

== system DSR_delay_beta_test/DSR_Input2/(I-beta*K)V_dot_est/DerivativeEstimate1/Derivative Estimator/DSRdelay ==
  Input : Inport
  Gain : Gain  Gain=2
  Sum : Sum  Inputs=-++
  Transport Delay1 : TransportDelay  DelayTime=2*delay
  Transport Delay2 : TransportDelay  DelayTime=delay
  Out1 : Outport
  wires:
  Input/1 -> Transport Delay2/1, Transport Delay1/1, Sum/2
  Transport Delay2/1 -> Gain/1
  Transport Delay1/1 -> Sum/3
  Gain/1 -> Sum/1
  Sum/1 -> Out1/1

== system DSR_delay_beta_test/DSR_Input2/(I-beta*K)V_dot_est/DerivativeEstimate1/Derivative Estimator1/DSRdelay ==
  Input : Inport
  Gain : Gain  Gain=2
  Sum : Sum  Inputs=-++
  Transport Delay1 : TransportDelay  DelayTime=2*delay
  Transport Delay2 : TransportDelay  DelayTime=delay
  Out1 : Outport
  wires:
  Input/1 -> Transport Delay2/1, Transport Delay1/1, Sum/2
  Transport Delay2/1 -> Gain/1
  Transport Delay1/1 -> Sum/3
  Gain/1 -> Sum/1
  Sum/1 -> Out1/1

== system DSR_delay_beta_test/DSR_Input2/(I-beta*K)V_dot_est/DerivativeEstimate1/Derivative Estimator2/DSRdelay ==
  Input : Inport
  Gain : Gain  Gain=2
  Sum : Sum  Inputs=-++
  Transport Delay1 : TransportDelay  DelayTime=2*delay
  Transport Delay2 : TransportDelay  DelayTime=delay
  Out1 : Outport
  wires:
  Input/1 -> Transport Delay2/1, Transport Delay1/1, Sum/2
  Transport Delay2/1 -> Gain/1
  Transport Delay1/1 -> Sum/3
  Gain/1 -> Sum/1
  Sum/1 -> Out1/1

== system DSR_delay_beta_test/DSR_Input2/(I-beta*K)V_dot_est/DerivativeEstimate1/Derivative Estimator3/DSRdelay ==
  Input : Inport
  Gain : Gain  Gain=2
  Sum : Sum  Inputs=-++
  Transport Delay1 : TransportDelay  DelayTime=2*delay
  Transport Delay2 : TransportDelay  DelayTime=delay
  Out1 : Outport
  wires:
  Input/1 -> Transport Delay2/1, Transport Delay1/1, Sum/2
  Transport Delay2/1 -> Gain/1
  Transport Delay1/1 -> Sum/3
  Gain/1 -> Sum/1
  Sum/1 -> Out1/1

== system DSR_delay_beta_test/DSR_Input2/(I-beta*K)V_dot_est/DerivativeEstimate1/Derivative Estimator4/DSRdelay ==
  Input : Inport
  Gain : Gain  Gain=2
  Sum : Sum  Inputs=-++
  Transport Delay1 : TransportDelay  DelayTime=2*delay
  Transport Delay2 : TransportDelay  DelayTime=delay
  Out1 : Outport
  wires:
  Input/1 -> Transport Delay2/1, Transport Delay1/1, Sum/2
  Transport Delay2/1 -> Gain/1
  Transport Delay1/1 -> Sum/3
  Gain/1 -> Sum/1
  Sum/1 -> Out1/1

== system DSR_delay_beta_test/DSR_Input2/(I-beta*K)V_dot_est/DerivativeEstimate1/Derivative Estimator5/DSRdelay ==
  Input : Inport
  Gain : Gain  Gain=2
  Sum : Sum  Inputs=-++
  Transport Delay1 : TransportDelay  DelayTime=2*delay
  Transport Delay2 : TransportDelay  DelayTime=delay
  Out1 : Outport
  wires:
  Input/1 -> Transport Delay2/1, Transport Delay1/1, Sum/2
  Transport Delay2/1 -> Gain/1
  Transport Delay1/1 -> Sum/3
  Gain/1 -> Sum/1
  Sum/1 -> Out1/1
